simulink model "RP20231104WLR_231105"  (R2018b)
settings: Solver=FixedStepDiscrete  StartTime=0.0  StopTime=10.0  FixedStep=0.0005  RelTol=1e-3  EnableMultiTasking=on
undefined symbols (not defined in the file or in its folder): I_AN06_5V, I_AN07_5V, I_AN08_5V, I_AN09_5V, I_HALL1, I_SW01_L, O_SW12_HS1A, O_SW14_HS1A, PWM3
libraries: ec5744lib x60, simulink x35, canmsglib x5
(part 2 of 2)

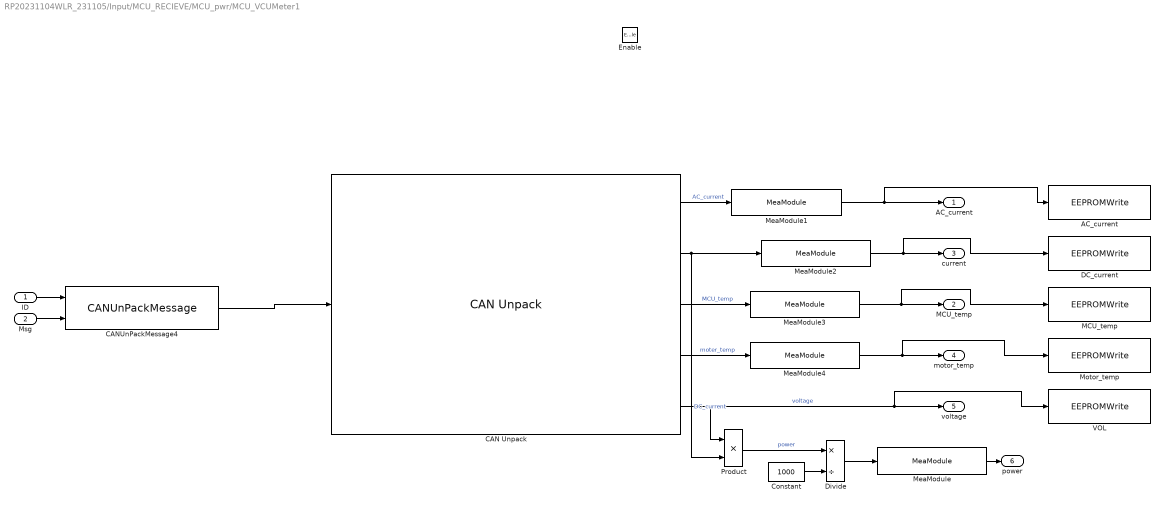
== system RP20231104WLR_231105/Input/MCU_RECIEVE/MCU_pwr/MCU_VCUMeter1 ==
  ID : Inport
  Msg : Inport  Port=2
  Enable : EnablePort
  AC_current : ec5744lib/RapidECU_U3/09MemoryManagement/EEPROMWrite  buffer=0  sampletime=-1
      settings: SourceProductName=ECUCoder for MPC5744
  CAN Unpack : canmsglib/CAN Unpack  CANdbFile=E:\candbc\MCU_No1.dbc  MsgList=(none)  MsgName=MCU2VCU2_ID1  MsgIDType=Extended (29-bit identifier)  MsgIdentifier=218089455  MsgLength=8  SignalInfo=MCU2VCU2_Current_AC_Feedback_ID1$48$16$1$2$1$0$1.000000e-01$-1600$-1600$1600$#MCU2VCU2_Current_DC_feedback_ID1$32$16$1$2$1$0$1.000000e-01$-1600$-1600$1600$#MCU2VCU2_MCU_Temp_ID1$0$8$1$2$1$0$1$-50$-50$200$#MCU2VCU2_Motor_Temp_ID1$8$8$1$2$1$0$1$-50$-50$200$#MCU2VCU2_Voltage_Feedback_ID1$16$16$1$2$1$0$1.000000e-01$0$0$1000$#  NSignals=5  IDPort=off  TimestampPort=off  ErrorPort=off  RemotePort=off  LengthPort=off  StatusPort=off  StartBits=str2num('[int32(48);int32(32);int32(0);int32(8);int32(16)]')  SignalSizes=str2num('[int32(16);int32(16);int32(8);int32(8);int32(16)]')  ByteOrders=str2num('[int32(1);int32(1);int32(1);int32(1);int32(1)]')  DataTypes=str2num('[int32(2);int32(2);int32(2);int32(2);int32(2)]')  MultiplexTypes=str2num('[int32(1);int32(1);int32(1);int32(1);int32(1)]')  MultiplexValues=str2num('[double(0);double(0);double(0);double(0);double(0)]')  Factors=str2num('[double(1.000000e-01);double(1.000000e-01);double(1);double(1);double(1.000000e-01)]')  Offsets=str2num('[double(-1600);double(-1600);double(-50);double(-50);double(0)]')  Minimums=str2num('[double(-1600);double(-1600);double(-50);double(-50);double(0)]')  Maximums=str2num('[double(1600);double(1600);double(200);double(200);double(1000)]')  ApplyMinMax=off
      settings: SourceProductBaseCode=XP,ME,VN  DataFormat=CANdb specified signals
  CANUnPackMessage4 : ec5744lib/RapidECU_U3/04CANCommunication/CANUnPackMessage  datalength=8  canmessagetype=Extended(29-bit ID)  sampletime=-1
      settings: SourceProductName=ECUCoder for MPC5744
  Constant : Constant  Value=1000
  DC_current : ec5744lib/RapidECU_U3/09MemoryManagement/EEPROMWrite  buffer=1  sampletime=-1
      settings: SourceProductName=ECUCoder for MPC5744
  Divide : Product  Inputs=*/
  "MCU_temp " : ec5744lib/RapidECU_U3/09MemoryManagement/EEPROMWrite  buffer=2  sampletime=-1
      settings: SourceProductName=ECUCoder for MPC5744
  MeaModule : ec5744lib/RapidECU_U3/07Calibration/MeaModule  signal=motor_power
      settings: SourceProductName=ECUCoder for MPC5744
  MeaModule1 : ec5744lib/RapidECU_U3/07Calibration/MeaModule  signal=AC_current
      settings: SourceProductName=ECUCoder for MPC5744
  MeaModule2 : ec5744lib/RapidECU_U3/07Calibration/MeaModule  signal=DC_current
      settings: SourceProductName=ECUCoder for MPC5744
  MeaModule3 : ec5744lib/RapidECU_U3/07Calibration/MeaModule  signal=MCU_Temp
      settings: SourceProductName=ECUCoder for MPC5744
  MeaModule4 : ec5744lib/RapidECU_U3/07Calibration/MeaModule  signal=motor_Temp
      settings: SourceProductName=ECUCoder for MPC5744
  Motor_temp : ec5744lib/RapidECU_U3/09MemoryManagement/EEPROMWrite  buffer=3  sampletime=-1
      settings: SourceProductName=ECUCoder for MPC5744
  Product : Product
  VOL : ec5744lib/RapidECU_U3/09MemoryManagement/EEPROMWrite  buffer=4  sampletime=-1
      settings: SourceProductName=ECUCoder for MPC5744
  "AC_current " : Outport  VectorParamsAs1DForOutWhenUnconnected=on
  MCU_temp : Outport  Port=2  VectorParamsAs1DForOutWhenUnconnected=on
  current : Outport  Port=3  VectorParamsAs1DForOutWhenUnconnected=on
  motor_temp : Outport  Port=4  VectorParamsAs1DForOutWhenUnconnected=on
  voltage : Outport  Port=5  VectorParamsAs1DForOutWhenUnconnected=on
  power : Outport  Port=6  VectorParamsAs1DForOutWhenUnconnected=on
  wires:
  Msg/1 -> CANUnPackMessage4/2
  ID/1 -> CANUnPackMessage4/1
  CANUnPackMessage4/1 -> CAN Unpack/1
  CAN Unpack/1 -> MeaModule1/1  "AC_current"
  CAN Unpack/5 -> Product/1, VOL/1, voltage/1  "voltage"
  CAN Unpack/4 -> MeaModule4/1  "moter_temp"
  MeaModule/1 -> power/1
  Product/1 -> Divide/1  "power"
  Constant/1 -> Divide/2
  Divide/1 -> MeaModule/1
  MeaModule1/1 -> AC_current/1, "AC_current "/1
  MeaModule2/1 -> DC_current/1, current/1
  CAN Unpack/3 -> MeaModule3/1  "MCU_temp"
  CAN Unpack/2 -> Product/2, MeaModule2/1  "DC_current"
  MeaModule3/1 -> "MCU_temp "/1, MCU_temp/1
  MeaModule4/1 -> Motor_temp/1, motor_temp/1

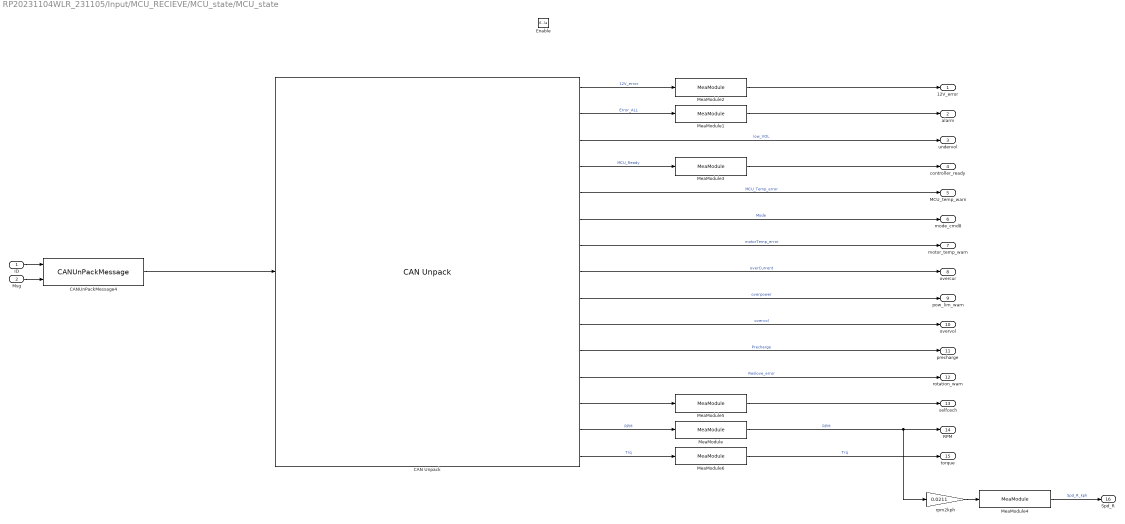
== system RP20231104WLR_231105/Input/MCU_RECIEVE/MCU_state/MCU_state ==
  ID : Inport
  Msg : Inport  Port=2
  Enable : EnablePort
  CAN Unpack : canmsglib/CAN Unpack  CANdbFile=E:\candbc\MCU_No1.dbc  MsgList=(none)  MsgName=MCU2VCU1_ID1  MsgIDType=Extended (29-bit identifier)  MsgIdentifier=218089199  MsgLength=8  SignalInfo=MCU2VCU1_12V_error_ID1$45$1$1$2$1$0$1$0$0$1$#MCU2VCU1_Error_All_ID1$56$2$1$2$1$0$1$0$0$3$#MCU2VCU1_LowVoltage_error_ID1$46$1$1$2$1$0$1$0$0$1$#MCU2VCU1_MCU_Ready_ID1$40$1$1$2$1$0$1$0$0$1$#MCU2VCU1_MCU_Temp_error_ID1$48$1$1$2$1$0$1$0$0$1$#MCU2VCU1_Mode_Feedback_ID1$32$8$1$2$1$0$1$0$0$255$#MCU2VCU1_MotorTemp_error_ID1$49$1$1$2$1$0$1$0$0$1$#MCU2VCU1_OverCurrent_error_ID1$43$1$1$2$1$0$1$0$0$1$#MCU2VCU1_OverPower_error_ID1$47$1$1$2$1$0$1$0$0$1$#MCU2VCU1_OverVoltage_error_ID1$44$1$1$2$1$0$1$0$0$1$#MCU2VCU1_PrechargeState_ID1$41$1$1$2$1$0$1$0$0$1$#MCU2VCU1_Reslove_Error_ID1$42$1$1$2$1$0$1$0$0$1$#MCU2VCU1_Selfcheck_ID1$55$1$1$2$1$0$1$0$0$1$#MCU2VCU1_Speed_Feedback_ID1$0$16$1$2$1$0$5.000000e-01$-10000$-10000$10000$#MCU2VCU1_Torque_Feedback_ID1$16$16$1$2$1$0$1$0$0$1000$#  NSignals=15  IDPort=off  TimestampPort=off  ErrorPort=off  RemotePort=off  LengthPort=off  StatusPort=off  StartBits=str2num('[int32(45);int32(56);int32(46);int32(40);int32(48);int32(32);int32(49);int32(43);int32(47);int32(44);int32(41);int32(42);int32(55);int32(0);int32(16)]')  SignalSizes=str2num('[int32(1);int32(2);int32(1);int32(1);int32(1);int32(8);int32(1);int32(1);int32(1);int32(1);int32(1);int32(1);int32(1);int32(16);int32(16)]')  ByteOrders=str2num('[int32(1);int32(1);int32(1);int32(1);int32(1);int32(1);int32(1);int32(1);int32(1);int32(1);int32(1);int32(1);int32(1);int32(1);int32(1)]')  DataTypes=str2num('[int32(2);int32(2);int32(2);int32(2);int32(2);int32(2);int32(2);int32(2);int32(2);int32(2);int32(2);int32(2);int32(2);int32(2);int32(2)]')  MultiplexTypes=str2num('[int32(1);int32(1);int32(1);int32(1);int32(1);int32(1);int32(1);int32(1);int32(1);int32(1);int32(1);int32(1);int32(1);int32(1);int32(1)]')  MultiplexValues=str2num('[double(0);double(0);double(0);double(0);double(0);double(0);double(0);double(0);double(0);double(0);double(0);double(0);double(0);double(0);double(0)]')  Factors=str2num('[double(1);double(1);double(1);double(1);double(1);double(1);double(1);double(1);double(1);double(1);double(1);double(1);double(1);double(5.000000e-01);double(1)]')  Offsets=str2num('[double(0);double(0);double(0);double(0);double(0);double(0);double(0);double(0);double(0);double(0);double(0);double(0);double(0);double(-10000);double(0)]')  Minimums=str2num('[double(0);double(0);double(0);double(0);double(0);double(0);double(0);double(0);double(0);double(0);double(0);double(0);double(0);double(-10000);double(0)]')  Maximums=str2num('[double(1);double(3);double(1);double(1);double(1);double(255);double(1);double(1);double(1);double(1);double(1);double(1);double(1);double(10000);double(1000)]')  ApplyMinMax=off
      settings: SourceProductBaseCode=XP,ME,VN  DataFormat=CANdb specified signals
  CANUnPackMessage4 : ec5744lib/RapidECU_U3/04CANCommunication/CANUnPackMessage  datalength=8  canmessagetype=Extended(29-bit ID)  sampletime=-1
      settings: SourceProductName=ECUCoder for MPC5744
  MeaModule : ec5744lib/RapidECU_U3/07Calibration/MeaModule  signal=RPM
      settings: SourceProductName=ECUCoder for MPC5744
  MeaModule1 : ec5744lib/RapidECU_U3/07Calibration/MeaModule  signal=alarm
      settings: SourceProductName=ECUCoder for MPC5744
  MeaModule2 : ec5744lib/RapidECU_U3/07Calibration/MeaModule  signal=L12V_error
      settings: SourceProductName=ECUCoder for MPC5744
  MeaModule3 : ec5744lib/RapidECU_U3/07Calibration/MeaModule  signal=controller_ready
      settings: SourceProductName=ECUCoder for MPC5744
  MeaModule4 : ec5744lib/RapidECU_U3/07Calibration/MeaModule  signal=Spd_R
      settings: SourceProductName=ECUCoder for MPC5744
  MeaModule5 : ec5744lib/RapidECU_U3/07Calibration/MeaModule  signal=selfcheck
      settings: SourceProductName=ECUCoder for MPC5744
  MeaModule6 : ec5744lib/RapidECU_U3/07Calibration/MeaModule  signal=trq
      settings: SourceProductName=ECUCoder for MPC5744
  rpm2kph : Gain  Gain=0.0211
  12V_error : Outport  VectorParamsAs1DForOutWhenUnconnected=on
  alarm : Outport  Port=2  VectorParamsAs1DForOutWhenUnconnected=on
  undervol : Outport  Port=3  VectorParamsAs1DForOutWhenUnconnected=on
  controller_ready : Outport  Port=4  VectorParamsAs1DForOutWhenUnconnected=on
  MCU_temp_warn : Outport  Port=5  VectorParamsAs1DForOutWhenUnconnected=on
  mode_cmd8 : Outport  Port=6  VectorParamsAs1DForOutWhenUnconnected=on
  motor_temp_warn : Outport  Port=7  VectorParamsAs1DForOutWhenUnconnected=on
  overcur : Outport  Port=8  VectorParamsAs1DForOutWhenUnconnected=on
  pow_lim_warn : Outport  Port=9  VectorParamsAs1DForOutWhenUnconnected=on
  overvol : Outport  Port=10  VectorParamsAs1DForOutWhenUnconnected=on
  precharge : Outport  Port=11  VectorParamsAs1DForOutWhenUnconnected=on
  rotation_warn : Outport  Port=12  VectorParamsAs1DForOutWhenUnconnected=on
  selfcech : Outport  Port=13  VectorParamsAs1DForOutWhenUnconnected=on
  RPM : Outport  Port=14  VectorParamsAs1DForOutWhenUnconnected=on
  torque : Outport  Port=15  VectorParamsAs1DForOutWhenUnconnected=on
  Spd_R : Outport  Port=16  VectorParamsAs1DForOutWhenUnconnected=on
  wires:
  Msg/1 -> CANUnPackMessage4/2
  ID/1 -> CANUnPackMessage4/1
  CANUnPackMessage4/1 -> CAN Unpack/1
  MeaModule/1 -> rpm2kph/1, RPM/1  "RPM"
  MeaModule1/1 -> alarm/1
  MeaModule2/1 -> 12V_error/1
  MeaModule3/1 -> controller_ready/1
  MeaModule5/1 -> selfcech/1
  MeaModule6/1 -> torque/1  "Trq"
  CAN Unpack/14 -> MeaModule/1  "RPM"
  CAN Unpack/15 -> MeaModule6/1  "Trq"
  CAN Unpack/13 -> MeaModule5/1
  CAN Unpack/11 -> precharge/1  "Precharge"
  CAN Unpack/10 -> overvol/1  "overvol"
  CAN Unpack/9 -> pow_lim_warn/1  "overpower"
  CAN Unpack/8 -> overcur/1  "overCurrent"
  CAN Unpack/7 -> motor_temp_warn/1  "motorTemp_error"
  CAN Unpack/6 -> mode_cmd8/1  "Mode"
  CAN Unpack/5 -> MCU_temp_warn/1  "MCU_Temp_error"
  CAN Unpack/4 -> MeaModule3/1  "MCU_Ready"
  CAN Unpack/3 -> undervol/1  "low_VOL"
  CAN Unpack/2 -> MeaModule1/1  "Error_ALL"
  CAN Unpack/1 -> MeaModule2/1  "12V_error"
  CAN Unpack/12 -> rotation_warn/1  "Reslove_error"
  rpm2kph/1 -> MeaModule4/1
  MeaModule4/1 -> Spd_R/1  "Spd_R_kph"

== stateflow chart RP20231104WLR_231105/drive_ready/Drive_ready/Chart1 ==
  state VehStat [parallel]
    settings: executionOrder=1
    state Guard
    state Standby
    state Trans
    state WaitForEngine
    state Init
    state Ready
    Standby -> Guard [order 1] : [KeyPressed&&Brk&&ACC_Release]
    Guard -> Trans [order 1] : after(0.25,sec){send(EbeepON,BeeperStat)}
    WaitForEngine -> Standby : [MCUReady]
    Trans -> Ready : after(2.5,sec){send(EbeepOFF,BeeperStat)}
    Standby -> WaitForEngine [order 2] : [~MCUReady]
    Guard -> Standby [order 2] : [~KeyPressed||~Brk||~ACC_Release]
    Init -> WaitForEngine : [after(1,sec)]
    Ready -> WaitForEngine : [~MCUReady]
    Guard -> WaitForEngine [order 3] : [~MCUReady]
    (default) -> Init
  state Output [parallel]
    du:
    VehReady = in(VehStat.Ready);
    VehStandby = in(VehStat.Standby)
    BeeperStOut = in(BeeperStat.ON);
    settings: executionOrder=3
  state BeeperStat [parallel]
    settings: executionOrder=2
    state OFF
    state ON
    (default) -> OFF
    OFF -> ON : EbeepON
    ON -> OFF : EbeepOFF
  data: Brk input boolean size=1; KeyPressed input boolean size=1; MCUReady input boolean size=1; VehReady output boolean size=1; BeeperStOut output boolean size=1; VehStandby output boolean; ACC_Release input boolean
  events: EbeepON local FUNCTION_CALL_EVENT; EbeepOFF local FUNCTION_CALL_EVENT
